simulink model "assign1_sim"  (R2022a)
settings: Solver=ode4  StartTime=0.0  StopTime=30  FixedStep=0.01  RelTol=1e-3
undefined symbols (not defined in the file): b, g, J, L, m, M, theta_d
libraries: fuzblock x1
settings Model: Creator=khan  LastModifiedBy=khan
settings SolverCC: AlgebraicLoopSolver=LineSearch
settings DebuggingCC: UnconnectedInputMsg=warning  UnconnectedOutputMsg=warning  UnconnectedLineMsg=warning  SFMachineParentedDataDiag=warning

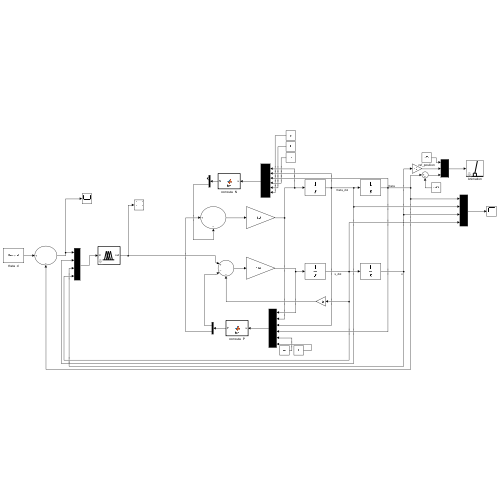
[thumbnail: Simulink's stored preview of the top-level diagram]
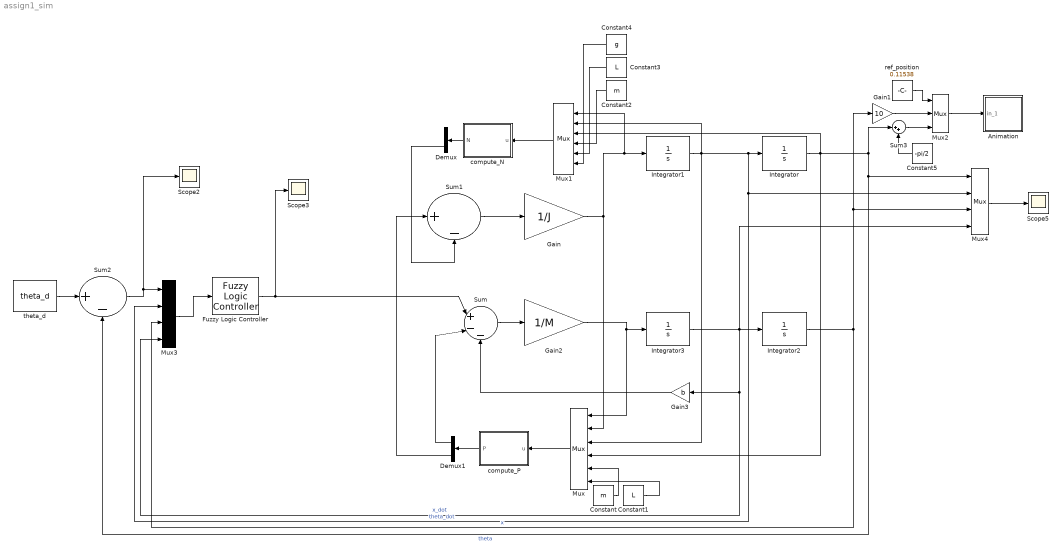
== system assign1_sim ==
  Animation : Subsystem  mask(Pendulum plot){RefBlock=ref_position}
      mask prompts: RefBlock "DC reference signal block name:"
      mask help: Pendulum plot
      mask Help: Pendulum animation function using Handle graphics.
      mask Display: plot([-10 10],[0 0],[-2 -2 2 2],[0 1 1 0],[0 3],[1 5])
  Constant : Constant  Value=m
  Constant1 : Constant  Value=L
  Constant2 : Constant  Value=m
  Constant3 : Constant  Value=L
  Constant4 : Constant  Value=g
  Constant5 : Constant  Value=-pi/2
  Demux : Demux  Outputs=2
  Demux1 : Demux  Outputs=2
  Fuzzy Logic Controller : fuzblock/Fuzzy Logic  Controller  FIS='IP_FIS.fis'  OutputSampleNumber=101  DataType=double  FuzzifiedInputs=off  RuleFiringStrengths=off  RuleOutputs=off  AggregatedOutputs=off  SimulateUsing=Interpreted execution  OutOfRangeInputValueMessage=warning  NoRuleFiredMessage=warning  EmptyOutputFuzzySetMessage=warning
  Gain : Gain  Gain=1/J
  Gain1 : Gain  Gain=10
  Gain2 : Gain  Gain=1/M
  Gain3 : Gain  Gain=b
  Integrator : Integrator  InitialCondition=pi/2-pi/20
  Integrator1 : Integrator
  Integrator2 : Integrator
  Integrator3 : Integrator
  Mux : Mux  Inputs=6
  Mux1 : Mux  Inputs=6
  Mux2 : Mux  Inputs=3
  Mux3 : Mux
  Mux4 : Mux
  Scope2 : Scope
  Scope3 : Scope
  Scope5 : Scope
  Sum : Sum  Inputs=|+--
  Sum1 : Sum  Inputs=|+-
  Sum2 : Sum  Inputs=|+-
  Sum3 : Sum  Inputs=|++
  compute_N : MATLAB Function  TreatAsAtomicUnit=on
  compute_P : MATLAB Function  TreatAsAtomicUnit=on
  ref_position : Constant  Value=0.11538
  theta_d : Constant  Value=theta_d
  wires:
  Integrator1/1 -> Mux1/2, Mux/3, Mux3/2, Mux4/2, Integrator/1  "theta_dot"
  Integrator3/1 -> Mux4/4, Mux3/4, Gain3/1, Integrator2/1  "x_dot"
  Integrator/1 -> Mux/4, Sum2/2, Mux4/1, Sum3/1, Mux1/3  "theta"
  Integrator2/1 -> Gain1/1, Mux4/3, Mux3/3  "x"
  Sum/1 -> Gain2/1
  Mux/1 -> compute_P/1(u)
  Sum1/1 -> Gain/1
  Constant/1 -> Mux/5
  Constant1/1 -> Mux/6
  Mux1/1 -> compute_N/1(u)
  Constant2/1 -> Mux1/4
  Constant3/1 -> Mux1/5
  Constant4/1 -> Mux1/6
  Gain/1 -> Mux1/1, Integrator1/1, Mux/2
  Gain2/1 -> Mux/1, Integrator3/1
  Gain3/1 -> Sum/3
  compute_N/1(N) -> Demux/1
  Demux/2 -> Sum1/2
  compute_P/1(P) -> Demux1/1
  Demux1/1 -> Sum/2
  Demux1/2 -> Sum1/1
  theta_d/1 -> Sum2/1
  Sum2/1 -> Mux3/1, Scope2/1
  Mux2/1 -> Animation/1(in_1)
  Sum3/1 -> Mux2/3
  Constant5/1 -> Sum3/2
  Gain1/1 -> Mux2/2
  ref_position/1 -> Mux2/1
  Mux3/1 -> Fuzzy Logic Controller/1
  Mux4/1 -> Scope5/1
  Fuzzy Logic Controller/1 -> Sum/1, Scope3/1

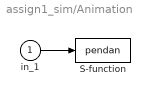
== system assign1_sim/Animation ==
  in_1 : Inport
  S-function : S-Function  FunctionName=pendan  Parameters=RefBlock  SFunctionDeploymentMode=off  EnableBusSupport=off
      settings: DeleteFcn=pendan([],[],[],'DeleteBlock');
  wires:
  in_1/1 -> S-function/1

== matlab function assign1_sim/compute_P ==
  data: u input; P output
function P = fcn(u)
P =zeros(2,1);
x_2dot= u(1);
theta_2dot= u(2);
theta_dot= u(3);
theta= u(4);
m= u(5);
L= u(6);
P(1)= m*(u(1)-L*u(2)*sin(u(4))-L*u(3)^2*cos(u(4)));
P(2)= P(1)*L*sin(u(4));
P=P;

== matlab function assign1_sim/compute_N ==
  data: u input; N output
function N = fcn(u)
N= zeros(2,1);
theta_2dot= u(1);
theta_dot= u(2);
theta= u(3);
m= u(4);
L= u(5);
g= u(6);
N(1)= m*(L*u(1)*cos(u(3))- L*u(2)^2*sin(u(3)) + g);
N(2)= N(1)*L*cos(u(3));
N= N;
